simulink model "testmodel4_smith"  (R2018b)
settings: Solver=VariableStepAuto  StartTime=0.0  StopTime=100  RelTol=1e-6
libraries: simulink x5
settings Model: Creator=Khor Jia Wei  LastModifiedBy=Khor Jia Wei
settings SolverCC: ZeroCrossAlgorithm=Adaptive

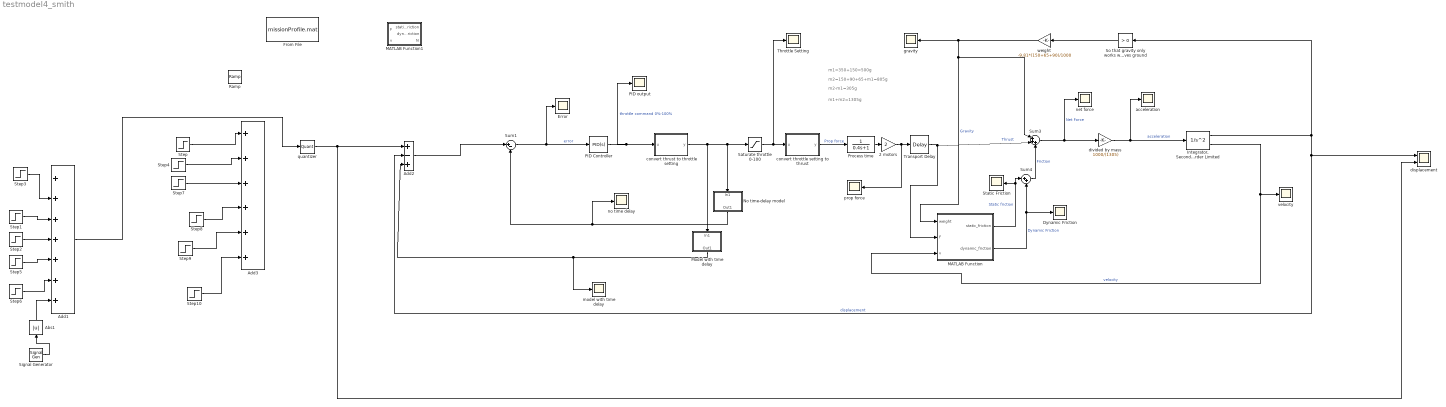
== system testmodel4_smith ==
  note: m1+m2=1305g
  note: m2-m1=305g
  note: m2=150+90+65+m1=805g
  note: m1=350+150=500g
  2 motors : Gain  Gain=2
  Abs1 : Abs
  Add1 : Sum  Inputs=+++++++
  Add2 : Sum  Inputs=+-+
  Add3 : Sum  Inputs=++++++
  Dynamic Friction : Scope
  Error : Scope
  From File : FromFile  FileName=missionProfile.mat  SampleTime=0
  "Integrator, Second-Order Limited" : SecondOrderIntegrator  ICX=0  LimitX=on  LowerLimitX=0  ReinitDXDTwhenXreachesSaturation=on
  MATLAB Function : MATLAB Function  TreatAsAtomicUnit=on
  MATLAB Function1 : MATLAB Function  TreatAsAtomicUnit=on
  Model with time delay : Subsystem
  No time-delay model : Subsystem
  PID Controller : simulink/Continuous/PID Controller  Controller=PID  Form=Parallel  TimeDomain=Continuous-time  SampleTime=-1  IntegratorMethod=Forward Euler  FilterMethod=Forward Euler  ControllerParametersSource=internal  P=20  I=6  D=10  UseFilter=on  N=100  TunerSelectOption=Transfer Function Based (PID Tuner App)  InitialConditionSource=internal  InitialConditionForIntegrator=0  InitialConditionForFilter=0  DifferentiatorICPrevScaledInput=0  ExternalReset=none  TrackingMode=off  Kt=1  LimitOutput=off  UpperSaturationLimit=inf  LowerSaturationLimit=-inf  LinearizeAsGain=on  AntiWindupMode=none  Kb=1  POutMin=[]  POutMax=[]  IOutMin=[]  IOutMax=[]  DOutMin=[]  DOutMax=[]  NOutMin=[]  NOutMax=[]  SumOutMin=[]  SumOutMax=[]  SaturationOutMin=[]  SaturationOutMax=[]  PParamMin=[]  PParamMax=[]  IParamMin=[]  IParamMax=[]  DParamMin=[]  DParamMax=[]  NParamMin=[]  NParamMax=[]  KbParamMin=[]  KbParamMax=[]  KtParamMin=[]  KtParamMax=[]  KbOutMin=[]  KbOutMax=[]  KtOutMin=[]  KtOutMax=[]  IntegratorOutMin=[]  IntegratorOutMax=[]  FilterOutMin=[]  FilterOutMax=[]  SumI1OutMin=[]  SumI1OutMax=[]  SumI2OutMin=[]  SumI2OutMax=[]  SumI3OutMin=[]  SumI3OutMax=[]  SumI4OutMin=[]  SumI4OutMax=[]  SumDOutMin=[]  SumDOutMax=[]  DifferentiatorOutMin=[]  DifferentiatorOutMax=[]  FilterDiffOutCoefMin=[]  FilterDiffOutCoefMax=[]  ReciprocalOutMin=[]  ReciprocalOutMax=[]  SumDenOutMin=[]  SumDenOutMax=[]  SumNumOutMin=[]  SumNumOutMax=[]  DivideOutMin=[]  DivideOutMax=[]  IntegratorContinuousStateAttributes=''  IntegratorStateMustResolveToSignalObject=off  IntegratorRTWStateStorageClass=Auto  FilterContinuousStateAttributes=''  FilterStateMustResolveToSignalObject=off  FilterRTWStateStorageClass=Auto  ParallelPVariant=InternalParameters  IdealPVariant=Disabled  IVariant=InternalParameters  DVariant=InternalParameters  IntegratorVariant=Continuous  SatVariant=Disabled  AWVariant=Passthrough  PCopyVariant=Disabled  TRVariant=Disabled  FdbkBlocksVariant=Forward  IdealPFdbkVariant=Disabled  SatFdbkVariant=Disabled  DerivativeFilterVariant=ContFilter  NVariant=InternalParameters  NCopyVariant=Disabled  FilterICVariant=InternalICsFilter  IntegratorICVariant=InternalICs  ExternalResetVariant=Disabled  TRSumVariant=Passthrough  SumFdbkVariant=Disabled  SumVariant=Sum_PID
  PID output : Scope
  "Process time  " : TransferFcn  Denominator=[0.4 1]
  Ramp : simulink/Sources/Ramp  slope=1  start=0  InitialOutput=0
  Saturate throttle 0-100 : Saturate  UpperLimit=100  LowerLimit=0
  Signal Generator : SignalGenerator  Amplitude=2  Frequency=0.2  Units=rad/sec
  So that gravity only works when the duocopter leaves ground : simulink/Logic and Bit Operations/Compare To Zero  relop=>  OutDataTypeStr=boolean
  Static Friction : Scope
  Step : Step  Time=0.5  After=0.5  SampleTime=0
  Step1 : Step  Time=7  After=0.3  SampleTime=0
  Step10 : Step  Time=32  After=2  SampleTime=0
  Step2 : Step  Time=9  After=0.2  SampleTime=0
  Step3 : Step  Time=5  After=-0.2  SampleTime=0
  Step4 : Step  After=0.5  SampleTime=0
  Step5 : Step  Time=15  After=-0.5  SampleTime=0
  Step6 : Step  Time=25  After=1.4  SampleTime=0
  Step7 : Step  Time=20  SampleTime=0
  Step8 : Step  Time=25  After=-0.5  SampleTime=0
  Step9 : Step  Time=27  After=-1  SampleTime=0
  Sum1 : Sum  Inputs=|+-
  Sum3 : Sum  Inputs=|+++
  Sum4 : Sum  Inputs=|++
  Throttle Setting : Scope
  Transport Delay : TransportDelay  DelayTime=0.6
  acceleration : Scope
  convert throttle setting to thrust : MATLAB Function  TreatAsAtomicUnit=on
  convert thrust to throttle setting : MATLAB Function  TreatAsAtomicUnit=on
  displacement : Scope  NumInputPorts=2
  divided by mass : Gain  Gain=1000/(1305)
  gravity : Scope
  model with time delay : Scope
  net force : Scope
  no time delay : Scope
  prop force : Scope
  quantizer : Quantizer
  velocity : Scope
  weight : Gain  Gain=-9.81*(150+65+90)/1000
  wires:
  So that gravity only works when the duocopter leaves ground/1 -> weight/1
  weight/1 -> MATLAB Function/1(weight), Sum3/1, gravity/1  "Gravity"
  Step5/1 -> Add1/5
  Sum1/1 -> PID Controller/1, Error/1  "error"
  quantizer/1 -> displacement/2, Add2/1
  Step2/1 -> Add1/4
  Step1/1 -> Add1/3
  divided by mass/1 -> "Integrator, Second-Order Limited"/1, acceleration/1  "acceleration"
  "Integrator, Second-Order Limited"/1 -> displacement/1, Add2/2, So that gravity only works when the duocopter leaves ground/1  "displacement"
  "Integrator, Second-Order Limited"/2 -> MATLAB Function/3(v), velocity/1  "velocity"
  PID Controller/1 -> PID output/1, convert thrust to throttle setting/1(u)  "throttle command 0%-100%"
  Sum3/1 -> divided by mass/1, net force/1  "Net Force"
  MATLAB Function/1(static_friction) -> Static Friction/1, Sum4/1  "Static friction"
  MATLAB Function/2(dynamic_friction) -> Dynamic Friction/1, Sum4/2  "Dynamic Friction"
  2 motors/1 -> prop force/1, Transport Delay/1
  Signal Generator/1 -> Abs1/1
  Add2/1 -> Sum1/1
  Model with time delay/1(Out1) -> model with time delay/1, Add2/3
  No time-delay model/1(Out1) -> no time delay/1, Sum1/2
  convert thrust to throttle setting/1(y) -> Saturate throttle 0-100/1, No time-delay model/1(In1), Model with time delay/1(In1)
  Saturate throttle 0-100/1 -> convert throttle setting to thrust/1(u), Throttle Setting/1
  Step6/1 -> Add1/6
  Sum4/1 -> Sum3/3  "Friction"
  Transport Delay/1 -> Sum3/2, MATLAB Function/2(F)  "Thrust"
  Abs1/1 -> Add1/7
  Step/1 -> Add3/1
  Step4/1 -> Add3/2
  Step7/1 -> Add3/3
  Step3/1 -> Add1/2
  Step8/1 -> Add3/4
  Step9/1 -> Add3/5
  Step10/1 -> Add3/6
  Add1/1 -> quantizer/1
  convert throttle setting to thrust/1(y) -> "Process time  "/1  "Prop force"
  "Process time  "/1 -> 2 motors/1

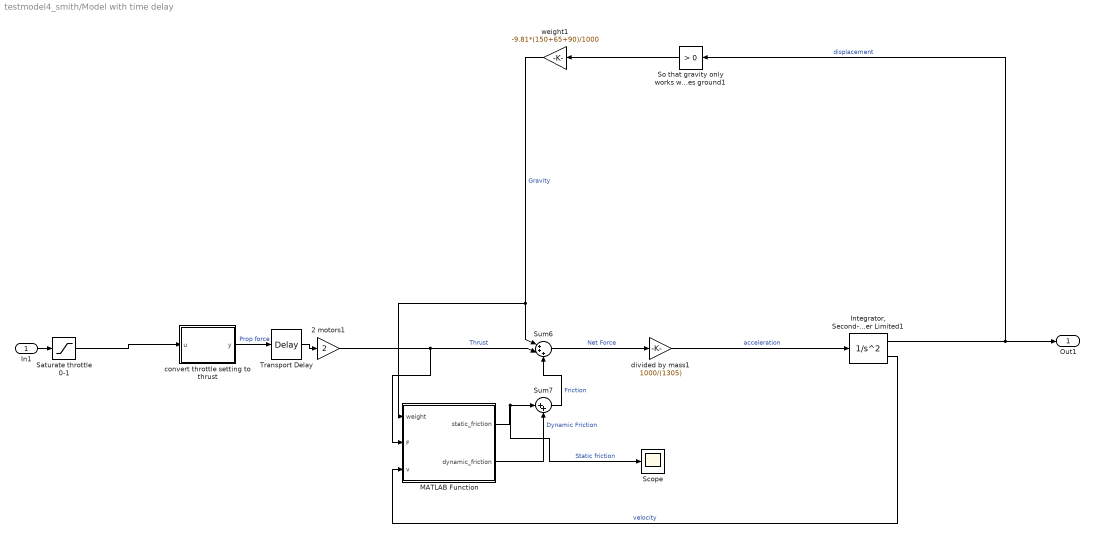
== system testmodel4_smith/Model with time delay ==
  In1 : Inport
  2 motors1 : Gain  Gain=2
  "Integrator, Second-Order Limited1" : SecondOrderIntegrator  ICX=0  LimitX=on  LowerLimitX=0  ReinitDXDTwhenXreachesSaturation=on
  MATLAB Function : MATLAB Function  TreatAsAtomicUnit=on
  Saturate throttle 0-1 : Saturate  UpperLimit=100  LowerLimit=0
  Scope : Scope
  So that gravity only works when the duocopter leaves ground1 : simulink/Logic and Bit Operations/Compare To Zero  relop=>  OutDataTypeStr=boolean
  Sum6 : Sum  Inputs=|+++
  Sum7 : Sum  Inputs=|++
  Transport Delay : TransportDelay  DelayTime=0.8
  convert throttle setting to thrust : MATLAB Function  TreatAsAtomicUnit=on
  divided by mass1 : Gain  Gain=1000/(1305)
  weight1 : Gain  Gain=-9.81*(150+65+90)/1000
  Out1 : Outport
  wires:
  "Integrator, Second-Order Limited1"/2 -> MATLAB Function/3(v)  "velocity"
  divided by mass1/1 -> "Integrator, Second-Order Limited1"/1  "acceleration"
  Transport Delay/1 -> 2 motors1/1
  Saturate throttle 0-1/1 -> convert throttle setting to thrust/1(u)
  So that gravity only works when the duocopter leaves ground1/1 -> weight1/1
  2 motors1/1 -> MATLAB Function/2(F), Sum6/2  "Thrust"
  MATLAB Function/1(static_friction) -> Scope/1, Sum7/1  "Static friction"
  Sum6/1 -> divided by mass1/1  "Net Force"
  "Integrator, Second-Order Limited1"/1 -> Out1/1, So that gravity only works when the duocopter leaves ground1/1  "displacement"
  MATLAB Function/2(dynamic_friction) -> Sum7/2  "Dynamic Friction"
  In1/1 -> Saturate throttle 0-1/1
  convert throttle setting to thrust/1(y) -> Transport Delay/1  "Prop force"
  Sum7/1 -> Sum6/3  "Friction"
  weight1/1 -> MATLAB Function/1(weight), Sum6/1  "Gravity"

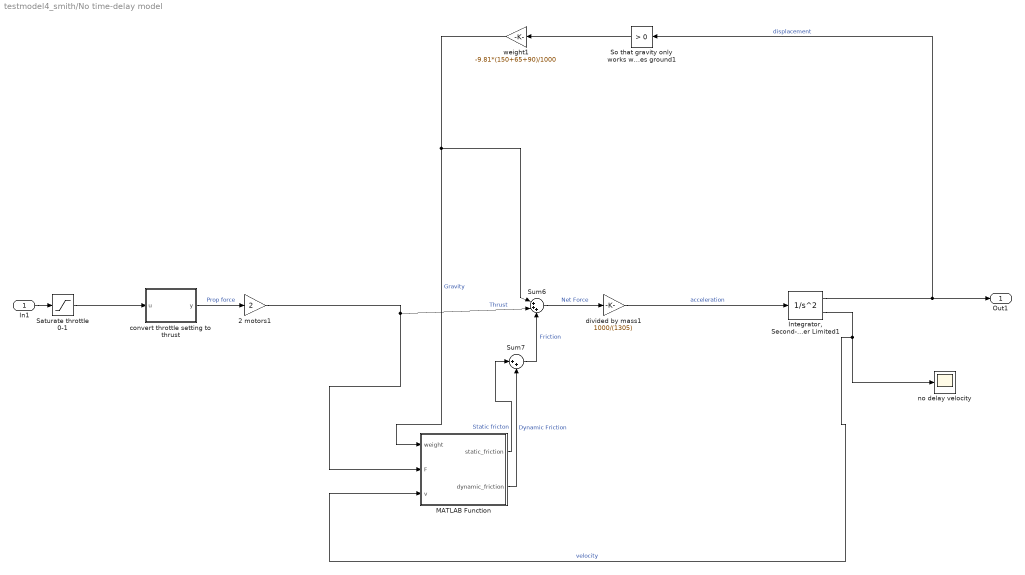
== system testmodel4_smith/No time-delay model ==
  In1 : Inport
  2 motors1 : Gain  Gain=2
  "Integrator, Second-Order Limited1" : SecondOrderIntegrator  ICX=0  LimitX=on  LowerLimitX=0  ReinitDXDTwhenXreachesSaturation=on
  MATLAB Function : MATLAB Function  TreatAsAtomicUnit=on
  Saturate throttle 0-1 : Saturate  UpperLimit=100  LowerLimit=0
  So that gravity only works when the duocopter leaves ground1 : simulink/Logic and Bit Operations/Compare To Zero  relop=>  OutDataTypeStr=boolean
  Sum6 : Sum  Inputs=|+++
  Sum7 : Sum  Inputs=|++
  convert throttle setting to thrust : MATLAB Function  TreatAsAtomicUnit=on
  divided by mass1 : Gain  Gain=1000/(1305)
  no delay velocity : Scope
  weight1 : Gain  Gain=-9.81*(150+65+90)/1000
  Out1 : Outport
  wires:
  divided by mass1/1 -> "Integrator, Second-Order Limited1"/1  "acceleration"
  2 motors1/1 -> MATLAB Function/2(F), Sum6/2  "Thrust"
  weight1/1 -> MATLAB Function/1(weight), Sum6/1  "Gravity"
  So that gravity only works when the duocopter leaves ground1/1 -> weight1/1
  "Integrator, Second-Order Limited1"/1 -> Out1/1, So that gravity only works when the duocopter leaves ground1/1  "displacement"
  "Integrator, Second-Order Limited1"/2 -> MATLAB Function/3(v), no delay velocity/1  "velocity"
  Saturate throttle 0-1/1 -> convert throttle setting to thrust/1(u)
  In1/1 -> Saturate throttle 0-1/1
  Sum6/1 -> divided by mass1/1  "Net Force"
  convert throttle setting to thrust/1(y) -> 2 motors1/1  "Prop force"
  MATLAB Function/2(dynamic_friction) -> Sum7/2  "Dynamic Friction"
  MATLAB Function/1(static_friction) -> Sum7/1  "Static fricton"
  Sum7/1 -> Sum6/3  "Friction"

== matlab function testmodel4_smith/No time-delay model/MATLAB Function ==
  data: weight input; F input; static_friction output; dynamic_friction output; v input
function [static_friction,dynamic_friction]=stickslip(weight,F,v)

%F=T-mg
%v=velocity
weight=double(weight);
%% mass inputs
m_carriage=350/1000; %in kg, given by errikos
m_motorprop=45/1000; %in kg, per motor prop
m_cw=150/1000; %estimated, errikos said 100 to 200g
m_arm=65/1000; 
m_wires=m_cw+150/1000; 
m1=m_carriage+m_cw;
m2=m_arm+2*m_motorprop+m_wires+m_carriage;

%% moment arm lengths

x1=11.5/1000; %in mm, from thrust to edge of arm
x2=10.59/1000; %from cg of arm to edge of arm
h=210.4/1000; %height of carriage
x3=35.8/1000; %thickness of carriage

%% Estimated Tension Force 
tension=m1*(9.81-(F+(m1-m2)*9.81)/(m1+m2));

%% Moment balance to obtain N, and friction
mu_dyn=0.17; %mu_dyn is between 0.11 to 0.17
N2=(F*(x1+x3)-(m2-m1-150/1000)*9.81*(x3+x2)-(m1+150/1000)*9.81*(x3/2)+tension*(x3/2))/h; %Normal contact force on carraige 2
f2=2*mu_dyn*N2; %friction of cart 2
N1=(m_cw*9.81*x3+m_carriage*9.81*(x3/2)-tension*(x3/2))/h; %N of cart 1
f1=2*mu_dyn*N1; %friction of cart 1
max_static_friction=0.130*9.81; 

if abs(v)<1e-5 %we are stuck
    if abs(F+weight)>max_static_friction %we are unstuck
        dynamic_friction=-1*sign(v)*(f1+f2); %dynamic friction
        static_friction=0;
    else
        static_friction=-1*(F+weight); %static friction
        dynamic_friction=0;
    end
else %we are unstuck
    dynamic_friction=-1*sign(v)*(f1+f2);
    static_friction=0;
end

== matlab function testmodel4_smith/MATLAB Function ==
  data: weight input; F input; static_friction output; dynamic_friction output; v input
function [static_friction,dynamic_friction]=stickslip(weight,F,v)

%F=T-mg
%v=velocity
weight=double(weight);
%% mass inputs
m_carriage=350/1000; %in kg, given by errikos
m_motorprop=45/1000; %in kg, per motor prop
m_cw=150/1000; %estimated, errikos said 100 to 200g
m_arm=65/1000; 
m_wires=m_cw+150/1000; 
m1=m_carriage+m_cw;
m2=m_arm+2*m_motorprop+m_wires+m_carriage;

%% moment arm lengths

x1=11.5/1000; %in mm, from thrust to edge of arm
x2=10.59/1000; %from cg of arm to edge of arm
h=210.4/1000; %height of carriage
x3=35.8/1000; %thickness of carriage

%% Estimated Tension Force 
tension=m1*(9.81-(F+(m1-m2)*9.81)/(m1+m2));

%% Moment balance to obtain N, and friction
mu_dyn=0.17; %mu_dyn is between 0.11 to 0.17
N2=(F*(x1+x3)-(m2-m1-150/1000)*9.81*(x3+x2)-(m1+150/1000)*9.81*(x3/2)+tension*(x3/2))/h; %Normal contact force on carraige 2
f2=2*mu_dyn*N2; %friction of cart 2
N1=(m_cw*9.81*(x3)+m_carriage*9.81*(x3/2)-tension*(x3/2))/h; %N of cart 1
f1=2*mu_dyn*N1; %friction of cart 1
max_static_friction=0.130*9.81; 

if abs(v)<1e-5 %we are stuck
    if abs(F+weight)>max_static_friction %we are unstuck
        dynamic_friction=-1*sign(v)*(f1+f2); %dynamic friction
        static_friction=0;
    else
        static_friction=-1*(F+weight); %static friction
        dynamic_friction=0;
    end
else %we are unstuck
    dynamic_friction=-1*sign(v)*(f1+f2);
    static_friction=0;
end

== matlab function testmodel4_smith/convert throttle setting to thrust ==
  data: u input; y output
function y = throttle2thrust(u)
breakpoints1=[0,0.0663455814708608,0.720926457059366,1.46901888630337,2.12359976189187,2.14485238772267,2.45089019968613,2.77150124079070,3.22236051734401,3.63536987932247,3.71329617403539,4.37956599383083,4.38346230856648,5.04371055104320,5.64586828291574,5.86406190811191,5.88410009818094,6.00432923859516,7.26673521294442,7.82780453487743,7.94256871436372,7.96807186536068,8.50363803629673,8.65382325883435,8.80967584826018,10.0253260457817,10.0720818226094,10.0933344484402,10.8201742518534,11.4747551274419,12.3163591103414,12.9709399859299,14.3736132907624,15.0281941663509,15.8631187525608,16.5243790248390,17.2724714540830,17.9270523296715,17.9604493131199,18.7219005357432,18.7619769158813,19.4232371881595,20.8259104929920,21.5856918664429,21.5895881811786,22.1818280209968,22.2285837978245,22.2498364236553,22.2636506304453,22.9766762270685,23.7403539152551,24.3793495319010,24.3949347908436,25.0940449776966,25.1274419611450,25.1486945869758,25.8032754625643,25.8287786135613,26.4299243156324,26.7638941501163,28.0263001244656,28.6808810000541,29.5224849829536,30.1770658585421,30.8103941082998,30.8316467341306,30.8650437175790,31.5797391633746,32.2343200389631,32.2677170224115,33.0759240218626,34.4785973266951,35.9280264083554,36.6293630607716,37.2839439363601,38.0320363656042,38.6866172411927,39.4814654472644,40.1828020996807,41.5854754045132,42.3548204595880,42.3803236105849,42.9146753457592,43.2686833703122,44.4843335678337,45.9337626494940,46.5883435250825,48.0377726067427,48.8326208128145,49.4872016884030,50.1885383408193,50.2041235997618,50.2703609502678,50.2820498944748,50.3154468779232,50.5158287786135,51.6847231993073,53.0406407273120,53.8354889333838,55.8927431138048,55.9139957396356,55.9394988906326,56.5005682125656,56.8559121164565,58.1370204015368,60.2877861356133,60.9423670112019,61.6748741815033,61.6904594404459,61.7060446993884,63.7689662466977,63.8412251745224,64.0750040586612,65.2438984793549,66.0387466854267,66.7400833378429,68.1427566426754,68.7973375182639,69.5921857243357,69.6389415011634,70.2935223767519,71.0416148059960,71.6728177931706,71.6961956815845,71.7174483074152,72.4209102224146,72.4655407366593,73.1923805400725,75.2496347204935,75.9743492613236,75.9977271497375,76.0094160939444,76.0189797755683,77.4939120082255,78.1484928838140,79.5628551328535,79.5979219654743,80.3226365063044,80.3927701715460,80.4395259483738,81.6551761458953,81.7019319227230,81.7231845485538,81.7299853888197,83.1513610043833,84.6007900860436,86.0034633908761,86.7181588366717,86.7515558201201,86.7728084459509,86.7983115969478,87.0788462579143,87.3126251420531,87.3406786081497,87.6866713566751,89.5569024297851,90.3049948590291,90.6322852968234,91.0530872882731,91.8011797175171,92.4713458520482,93.2506087991774,93.9519454515937,95.3546187564262,96.1182964446128,96.7572920612587,97.0845824990529,97.5053844905027,98.2534769197467,98.9080577953352,99.9032879020973,99.9579375113765,100.263975323339];
breakpoints2=[0,0.0164109572459205,0.234387537524814,0.440340894785261,0.434997240110396,0.513532770937965,0.452809422359948,0.524567070851000,0.537639940323439,0.626181329588921,0.548995206507528,0.590408530237738,0.673086742846075,0.703961192078633,0.724445201665616,0.814842026582094,0.658158437722640,0.743147993027647,0.829091772381737,0.912363724398392,0.832208904275407,0.959625381300537,0.981669306242101,0.903457633273616,1.00854950854597,1.04061143659516,0.987174889846509,1.12708148497026,1.15460940299230,1.14422786943785,1.09271206967510,1.26428791519391,1.38530388139737,1.42624518229796,1.51085304798334,1.54710083886118,1.51441548443325,1.64824434706822,1.68658294886249,1.78124197453154,1.66505565431518,1.80475405510095,1.82327872464048,1.93767746513823,1.93834542197259,2.01144661792475,1.94992334043479,2.10059820937305,1.87154973853677,2.09028333656127,2.17762240352491,2.05056217014477,2.21324676802401,2.23911684224360,2.10622523967462,2.32211698498567,2.36292307523010,2.27713312835907,2.36599047180969,2.36405657773689,2.35871292306202,2.39611850578608,2.49453081271486,2.40502459691085,2.75155250612941,2.51786477146177,2.66737259547212,2.62233322035539,2.74003612066043,2.73363391344045,2.85389158959957,2.75147154166465,2.86814133539921,2.75147154166465,3.03599888787343,3.08500465428751,3.05873168546941,3.24433462450975,3.19321366145354,3.26446239045175,3.55552964130238,3.35619512903694,3.59411499194167,3.60289385319323,3.52563351268580,3.66915517116157,3.77976882293129,3.80862455817557,3.74450070207717,3.83213663874497,4.04908901854451,4.12508766280927,3.92217722001646,3.79036707136977,3.99412571331733,4.12924383866750,4.07847911925627,4.13245003147242,4.09940843339950,4.29329403718588,4.28547286988903,4.10573175809809,4.37986124291870,4.38146433932115,4.41780119111025,4.44229294170338,4.57989204958117,4.56421732920156,4.40016713068319,4.64935956035442,4.80594483522094,4.65969062605916,4.80254432770058,4.75177960828935,4.67857153924369,4.83460625574976,4.91253455309155,4.85954331089914,5.03766513339466,4.92366716699752,5.12583543552994,5.12761665375490,5.24205992470827,5.20509964654045,5.32330776510566,5.35427667288045,5.41949354925324,5.45625141625914,5.43309557933472,5.58316321478720,5.46204037549024,5.45834434767345,5.66530166429706,5.66447582675640,5.67534125792863,5.67569750157362,5.72165293177746,5.92471180942235,5.74758746913281,5.88196257202343,5.95570500653658,5.91046206362271,6.09279403828631,6.00807282235026,5.95677373747155,6.06008439451896,6.03514733936958,6.28731694807395,6.34507931051178,6.43478793747771,6.10292269282912,6.30143946400039,6.45106179489662,6.35968529995642,6.40296890282283,6.44749935844671,6.49737346874546,6.49113920495811,6.45106179489662,6.44838996755918,6.44126509465936,6.35220418341160,6.45907727690892,6.46709275892121,6.45373362223406,6.44571814022176,6.44838996755918,6.38604732968576,6.38028805742507,6.44037448554689,6.35541037621653,6.44644682040469,6.40831255749770];

if u<=breakpoints1(153)
    y=2.8E-06*u^3-0.00048*u^2+0.09*u+0.2;
else
    y=breakpoints2(153);
end

== matlab function testmodel4_smith/No time-delay model/convert throttle setting to thrust ==
  data: u input; y output
function y = throttle2thrust(u)
breakpoints1=[0,0.0663455814708608,0.720926457059366,1.46901888630337,2.12359976189187,2.14485238772267,2.45089019968613,2.77150124079070,3.22236051734401,3.63536987932247,3.71329617403539,4.37956599383083,4.38346230856648,5.04371055104320,5.64586828291574,5.86406190811191,5.88410009818094,6.00432923859516,7.26673521294442,7.82780453487743,7.94256871436372,7.96807186536068,8.50363803629673,8.65382325883435,8.80967584826018,10.0253260457817,10.0720818226094,10.0933344484402,10.8201742518534,11.4747551274419,12.3163591103414,12.9709399859299,14.3736132907624,15.0281941663509,15.8631187525608,16.5243790248390,17.2724714540830,17.9270523296715,17.9604493131199,18.7219005357432,18.7619769158813,19.4232371881595,20.8259104929920,21.5856918664429,21.5895881811786,22.1818280209968,22.2285837978245,22.2498364236553,22.2636506304453,22.9766762270685,23.7403539152551,24.3793495319010,24.3949347908436,25.0940449776966,25.1274419611450,25.1486945869758,25.8032754625643,25.8287786135613,26.4299243156324,26.7638941501163,28.0263001244656,28.6808810000541,29.5224849829536,30.1770658585421,30.8103941082998,30.8316467341306,30.8650437175790,31.5797391633746,32.2343200389631,32.2677170224115,33.0759240218626,34.4785973266951,35.9280264083554,36.6293630607716,37.2839439363601,38.0320363656042,38.6866172411927,39.4814654472644,40.1828020996807,41.5854754045132,42.3548204595880,42.3803236105849,42.9146753457592,43.2686833703122,44.4843335678337,45.9337626494940,46.5883435250825,48.0377726067427,48.8326208128145,49.4872016884030,50.1885383408193,50.2041235997618,50.2703609502678,50.2820498944748,50.3154468779232,50.5158287786135,51.6847231993073,53.0406407273120,53.8354889333838,55.8927431138048,55.9139957396356,55.9394988906326,56.5005682125656,56.8559121164565,58.1370204015368,60.2877861356133,60.9423670112019,61.6748741815033,61.6904594404459,61.7060446993884,63.7689662466977,63.8412251745224,64.0750040586612,65.2438984793549,66.0387466854267,66.7400833378429,68.1427566426754,68.7973375182639,69.5921857243357,69.6389415011634,70.2935223767519,71.0416148059960,71.6728177931706,71.6961956815845,71.7174483074152,72.4209102224146,72.4655407366593,73.1923805400725,75.2496347204935,75.9743492613236,75.9977271497375,76.0094160939444,76.0189797755683,77.4939120082255,78.1484928838140,79.5628551328535,79.5979219654743,80.3226365063044,80.3927701715460,80.4395259483738,81.6551761458953,81.7019319227230,81.7231845485538,81.7299853888197,83.1513610043833,84.6007900860436,86.0034633908761,86.7181588366717,86.7515558201201,86.7728084459509,86.7983115969478,87.0788462579143,87.3126251420531,87.3406786081497,87.6866713566751,89.5569024297851,90.3049948590291,90.6322852968234,91.0530872882731,91.8011797175171,92.4713458520482,93.2506087991774,93.9519454515937,95.3546187564262,96.1182964446128,96.7572920612587,97.0845824990529,97.5053844905027,98.2534769197467,98.9080577953352,99.9032879020973,99.9579375113765,100.263975323339];
breakpoints2=[0,0.0164109572459205,0.234387537524814,0.440340894785261,0.434997240110396,0.513532770937965,0.452809422359948,0.524567070851000,0.537639940323439,0.626181329588921,0.548995206507528,0.590408530237738,0.673086742846075,0.703961192078633,0.724445201665616,0.814842026582094,0.658158437722640,0.743147993027647,0.829091772381737,0.912363724398392,0.832208904275407,0.959625381300537,0.981669306242101,0.903457633273616,1.00854950854597,1.04061143659516,0.987174889846509,1.12708148497026,1.15460940299230,1.14422786943785,1.09271206967510,1.26428791519391,1.38530388139737,1.42624518229796,1.51085304798334,1.54710083886118,1.51441548443325,1.64824434706822,1.68658294886249,1.78124197453154,1.66505565431518,1.80475405510095,1.82327872464048,1.93767746513823,1.93834542197259,2.01144661792475,1.94992334043479,2.10059820937305,1.87154973853677,2.09028333656127,2.17762240352491,2.05056217014477,2.21324676802401,2.23911684224360,2.10622523967462,2.32211698498567,2.36292307523010,2.27713312835907,2.36599047180969,2.36405657773689,2.35871292306202,2.39611850578608,2.49453081271486,2.40502459691085,2.75155250612941,2.51786477146177,2.66737259547212,2.62233322035539,2.74003612066043,2.73363391344045,2.85389158959957,2.75147154166465,2.86814133539921,2.75147154166465,3.03599888787343,3.08500465428751,3.05873168546941,3.24433462450975,3.19321366145354,3.26446239045175,3.55552964130238,3.35619512903694,3.59411499194167,3.60289385319323,3.52563351268580,3.66915517116157,3.77976882293129,3.80862455817557,3.74450070207717,3.83213663874497,4.04908901854451,4.12508766280927,3.92217722001646,3.79036707136977,3.99412571331733,4.12924383866750,4.07847911925627,4.13245003147242,4.09940843339950,4.29329403718588,4.28547286988903,4.10573175809809,4.37986124291870,4.38146433932115,4.41780119111025,4.44229294170338,4.57989204958117,4.56421732920156,4.40016713068319,4.64935956035442,4.80594483522094,4.65969062605916,4.80254432770058,4.75177960828935,4.67857153924369,4.83460625574976,4.91253455309155,4.85954331089914,5.03766513339466,4.92366716699752,5.12583543552994,5.12761665375490,5.24205992470827,5.20509964654045,5.32330776510566,5.35427667288045,5.41949354925324,5.45625141625914,5.43309557933472,5.58316321478720,5.46204037549024,5.45834434767345,5.66530166429706,5.66447582675640,5.67534125792863,5.67569750157362,5.72165293177746,5.92471180942235,5.74758746913281,5.88196257202343,5.95570500653658,5.91046206362271,6.09279403828631,6.00807282235026,5.95677373747155,6.06008439451896,6.03514733936958,6.28731694807395,6.34507931051178,6.43478793747771,6.10292269282912,6.30143946400039,6.45106179489662,6.35968529995642,6.40296890282283,6.44749935844671,6.49737346874546,6.49113920495811,6.45106179489662,6.44838996755918,6.44126509465936,6.35220418341160,6.45907727690892,6.46709275892121,6.45373362223406,6.44571814022176,6.44838996755918,6.38604732968576,6.38028805742507,6.44037448554689,6.35541037621653,6.44644682040469,6.40831255749770];

if u<=breakpoints1(153)
    y=2.8E-06*u^3-0.00048*u^2+0.09*u+0.2;
else
    y=breakpoints2(153);
end

== matlab function testmodel4_smith/Model with time delay/convert throttle setting to thrust ==
  data: u input; y output
function y = throttle2thrust(u)
breakpoints1=[0,0.0663455814708608,0.720926457059366,1.46901888630337,2.12359976189187,2.14485238772267,2.45089019968613,2.77150124079070,3.22236051734401,3.63536987932247,3.71329617403539,4.37956599383083,4.38346230856648,5.04371055104320,5.64586828291574,5.86406190811191,5.88410009818094,6.00432923859516,7.26673521294442,7.82780453487743,7.94256871436372,7.96807186536068,8.50363803629673,8.65382325883435,8.80967584826018,10.0253260457817,10.0720818226094,10.0933344484402,10.8201742518534,11.4747551274419,12.3163591103414,12.9709399859299,14.3736132907624,15.0281941663509,15.8631187525608,16.5243790248390,17.2724714540830,17.9270523296715,17.9604493131199,18.7219005357432,18.7619769158813,19.4232371881595,20.8259104929920,21.5856918664429,21.5895881811786,22.1818280209968,22.2285837978245,22.2498364236553,22.2636506304453,22.9766762270685,23.7403539152551,24.3793495319010,24.3949347908436,25.0940449776966,25.1274419611450,25.1486945869758,25.8032754625643,25.8287786135613,26.4299243156324,26.7638941501163,28.0263001244656,28.6808810000541,29.5224849829536,30.1770658585421,30.8103941082998,30.8316467341306,30.8650437175790,31.5797391633746,32.2343200389631,32.2677170224115,33.0759240218626,34.4785973266951,35.9280264083554,36.6293630607716,37.2839439363601,38.0320363656042,38.6866172411927,39.4814654472644,40.1828020996807,41.5854754045132,42.3548204595880,42.3803236105849,42.9146753457592,43.2686833703122,44.4843335678337,45.9337626494940,46.5883435250825,48.0377726067427,48.8326208128145,49.4872016884030,50.1885383408193,50.2041235997618,50.2703609502678,50.2820498944748,50.3154468779232,50.5158287786135,51.6847231993073,53.0406407273120,53.8354889333838,55.8927431138048,55.9139957396356,55.9394988906326,56.5005682125656,56.8559121164565,58.1370204015368,60.2877861356133,60.9423670112019,61.6748741815033,61.6904594404459,61.7060446993884,63.7689662466977,63.8412251745224,64.0750040586612,65.2438984793549,66.0387466854267,66.7400833378429,68.1427566426754,68.7973375182639,69.5921857243357,69.6389415011634,70.2935223767519,71.0416148059960,71.6728177931706,71.6961956815845,71.7174483074152,72.4209102224146,72.4655407366593,73.1923805400725,75.2496347204935,75.9743492613236,75.9977271497375,76.0094160939444,76.0189797755683,77.4939120082255,78.1484928838140,79.5628551328535,79.5979219654743,80.3226365063044,80.3927701715460,80.4395259483738,81.6551761458953,81.7019319227230,81.7231845485538,81.7299853888197,83.1513610043833,84.6007900860436,86.0034633908761,86.7181588366717,86.7515558201201,86.7728084459509,86.7983115969478,87.0788462579143,87.3126251420531,87.3406786081497,87.6866713566751,89.5569024297851,90.3049948590291,90.6322852968234,91.0530872882731,91.8011797175171,92.4713458520482,93.2506087991774,93.9519454515937,95.3546187564262,96.1182964446128,96.7572920612587,97.0845824990529,97.5053844905027,98.2534769197467,98.9080577953352,99.9032879020973,99.9579375113765,100.263975323339];
breakpoints2=[0,0.0164109572459205,0.234387537524814,0.440340894785261,0.434997240110396,0.513532770937965,0.452809422359948,0.524567070851000,0.537639940323439,0.626181329588921,0.548995206507528,0.590408530237738,0.673086742846075,0.703961192078633,0.724445201665616,0.814842026582094,0.658158437722640,0.743147993027647,0.829091772381737,0.912363724398392,0.832208904275407,0.959625381300537,0.981669306242101,0.903457633273616,1.00854950854597,1.04061143659516,0.987174889846509,1.12708148497026,1.15460940299230,1.14422786943785,1.09271206967510,1.26428791519391,1.38530388139737,1.42624518229796,1.51085304798334,1.54710083886118,1.51441548443325,1.64824434706822,1.68658294886249,1.78124197453154,1.66505565431518,1.80475405510095,1.82327872464048,1.93767746513823,1.93834542197259,2.01144661792475,1.94992334043479,2.10059820937305,1.87154973853677,2.09028333656127,2.17762240352491,2.05056217014477,2.21324676802401,2.23911684224360,2.10622523967462,2.32211698498567,2.36292307523010,2.27713312835907,2.36599047180969,2.36405657773689,2.35871292306202,2.39611850578608,2.49453081271486,2.40502459691085,2.75155250612941,2.51786477146177,2.66737259547212,2.62233322035539,2.74003612066043,2.73363391344045,2.85389158959957,2.75147154166465,2.86814133539921,2.75147154166465,3.03599888787343,3.08500465428751,3.05873168546941,3.24433462450975,3.19321366145354,3.26446239045175,3.55552964130238,3.35619512903694,3.59411499194167,3.60289385319323,3.52563351268580,3.66915517116157,3.77976882293129,3.80862455817557,3.74450070207717,3.83213663874497,4.04908901854451,4.12508766280927,3.92217722001646,3.79036707136977,3.99412571331733,4.12924383866750,4.07847911925627,4.13245003147242,4.09940843339950,4.29329403718588,4.28547286988903,4.10573175809809,4.37986124291870,4.38146433932115,4.41780119111025,4.44229294170338,4.57989204958117,4.56421732920156,4.40016713068319,4.64935956035442,4.80594483522094,4.65969062605916,4.80254432770058,4.75177960828935,4.67857153924369,4.83460625574976,4.91253455309155,4.85954331089914,5.03766513339466,4.92366716699752,5.12583543552994,5.12761665375490,5.24205992470827,5.20509964654045,5.32330776510566,5.35427667288045,5.41949354925324,5.45625141625914,5.43309557933472,5.58316321478720,5.46204037549024,5.45834434767345,5.66530166429706,5.66447582675640,5.67534125792863,5.67569750157362,5.72165293177746,5.92471180942235,5.74758746913281,5.88196257202343,5.95570500653658,5.91046206362271,6.09279403828631,6.00807282235026,5.95677373747155,6.06008439451896,6.03514733936958,6.28731694807395,6.34507931051178,6.43478793747771,6.10292269282912,6.30143946400039,6.45106179489662,6.35968529995642,6.40296890282283,6.44749935844671,6.49737346874546,6.49113920495811,6.45106179489662,6.44838996755918,6.44126509465936,6.35220418341160,6.45907727690892,6.46709275892121,6.45373362223406,6.44571814022176,6.44838996755918,6.38604732968576,6.38028805742507,6.44037448554689,6.35541037621653,6.44644682040469,6.40831255749770];

if u<=breakpoints1(153)
    y=2.8E-06*u^3-0.00048*u^2+0.09*u+0.2;
else
    y=breakpoints2(153);
end

== matlab function testmodel4_smith/convert thrust to throttle setting ==
  data: u input; y output
function y = thrust2throttle(u)
breakpoints1=[0,0.0663455814708608,0.720926457059366,1.46901888630337,2.12359976189187,2.14485238772267,2.45089019968613,2.77150124079070,3.22236051734401,3.63536987932247,3.71329617403539,4.37956599383083,4.38346230856648,5.04371055104320,5.64586828291574,5.86406190811191,5.88410009818094,6.00432923859516,7.26673521294442,7.82780453487743,7.94256871436372,7.96807186536068,8.50363803629673,8.65382325883435,8.80967584826018,10.0253260457817,10.0720818226094,10.0933344484402,10.8201742518534,11.4747551274419,12.3163591103414,12.9709399859299,14.3736132907624,15.0281941663509,15.8631187525608,16.5243790248390,17.2724714540830,17.9270523296715,17.9604493131199,18.7219005357432,18.7619769158813,19.4232371881595,20.8259104929920,21.5856918664429,21.5895881811786,22.1818280209968,22.2285837978245,22.2498364236553,22.2636506304453,22.9766762270685,23.7403539152551,24.3793495319010,24.3949347908436,25.0940449776966,25.1274419611450,25.1486945869758,25.8032754625643,25.8287786135613,26.4299243156324,26.7638941501163,28.0263001244656,28.6808810000541,29.5224849829536,30.1770658585421,30.8103941082998,30.8316467341306,30.8650437175790,31.5797391633746,32.2343200389631,32.2677170224115,33.0759240218626,34.4785973266951,35.9280264083554,36.6293630607716,37.2839439363601,38.0320363656042,38.6866172411927,39.4814654472644,40.1828020996807,41.5854754045132,42.3548204595880,42.3803236105849,42.9146753457592,43.2686833703122,44.4843335678337,45.9337626494940,46.5883435250825,48.0377726067427,48.8326208128145,49.4872016884030,50.1885383408193,50.2041235997618,50.2703609502678,50.2820498944748,50.3154468779232,50.5158287786135,51.6847231993073,53.0406407273120,53.8354889333838,55.8927431138048,55.9139957396356,55.9394988906326,56.5005682125656,56.8559121164565,58.1370204015368,60.2877861356133,60.9423670112019,61.6748741815033,61.6904594404459,61.7060446993884,63.7689662466977,63.8412251745224,64.0750040586612,65.2438984793549,66.0387466854267,66.7400833378429,68.1427566426754,68.7973375182639,69.5921857243357,69.6389415011634,70.2935223767519,71.0416148059960,71.6728177931706,71.6961956815845,71.7174483074152,72.4209102224146,72.4655407366593,73.1923805400725,75.2496347204935,75.9743492613236,75.9977271497375,76.0094160939444,76.0189797755683,77.4939120082255,78.1484928838140,79.5628551328535,79.5979219654743,80.3226365063044,80.3927701715460,80.4395259483738,81.6551761458953,81.7019319227230,81.7231845485538,81.7299853888197,83.1513610043833,84.6007900860436,86.0034633908761,86.7181588366717,86.7515558201201,86.7728084459509,86.7983115969478,87.0788462579143,87.3126251420531,87.3406786081497,87.6866713566751,89.5569024297851,90.3049948590291,90.6322852968234,91.0530872882731,91.8011797175171,92.4713458520482,93.2506087991774,93.9519454515937,95.3546187564262,96.1182964446128,96.7572920612587,97.0845824990529,97.5053844905027,98.2534769197467,98.9080577953352,99.9032879020973,99.9579375113765,100.263975323339];
breakpoints2=[0,0.0164109572459205,0.234387537524814,0.440340894785261,0.434997240110396,0.513532770937965,0.452809422359948,0.524567070851000,0.537639940323439,0.626181329588921,0.548995206507528,0.590408530237738,0.673086742846075,0.703961192078633,0.724445201665616,0.814842026582094,0.658158437722640,0.743147993027647,0.829091772381737,0.912363724398392,0.832208904275407,0.959625381300537,0.981669306242101,0.903457633273616,1.00854950854597,1.04061143659516,0.987174889846509,1.12708148497026,1.15460940299230,1.14422786943785,1.09271206967510,1.26428791519391,1.38530388139737,1.42624518229796,1.51085304798334,1.54710083886118,1.51441548443325,1.64824434706822,1.68658294886249,1.78124197453154,1.66505565431518,1.80475405510095,1.82327872464048,1.93767746513823,1.93834542197259,2.01144661792475,1.94992334043479,2.10059820937305,1.87154973853677,2.09028333656127,2.17762240352491,2.05056217014477,2.21324676802401,2.23911684224360,2.10622523967462,2.32211698498567,2.36292307523010,2.27713312835907,2.36599047180969,2.36405657773689,2.35871292306202,2.39611850578608,2.49453081271486,2.40502459691085,2.75155250612941,2.51786477146177,2.66737259547212,2.62233322035539,2.74003612066043,2.73363391344045,2.85389158959957,2.75147154166465,2.86814133539921,2.75147154166465,3.03599888787343,3.08500465428751,3.05873168546941,3.24433462450975,3.19321366145354,3.26446239045175,3.55552964130238,3.35619512903694,3.59411499194167,3.60289385319323,3.52563351268580,3.66915517116157,3.77976882293129,3.80862455817557,3.74450070207717,3.83213663874497,4.04908901854451,4.12508766280927,3.92217722001646,3.79036707136977,3.99412571331733,4.12924383866750,4.07847911925627,4.13245003147242,4.09940843339950,4.29329403718588,4.28547286988903,4.10573175809809,4.37986124291870,4.38146433932115,4.41780119111025,4.44229294170338,4.57989204958117,4.56421732920156,4.40016713068319,4.64935956035442,4.80594483522094,4.65969062605916,4.80254432770058,4.75177960828935,4.67857153924369,4.83460625574976,4.91253455309155,4.85954331089914,5.03766513339466,4.92366716699752,5.12583543552994,5.12761665375490,5.24205992470827,5.20509964654045,5.32330776510566,5.35427667288045,5.41949354925324,5.45625141625914,5.43309557933472,5.58316321478720,5.46204037549024,5.45834434767345,5.66530166429706,5.66447582675640,5.67534125792863,5.67569750157362,5.72165293177746,5.92471180942235,5.74758746913281,5.88196257202343,5.95570500653658,5.91046206362271,6.09279403828631,6.00807282235026,5.95677373747155,6.06008439451896,6.03514733936958,6.28731694807395,6.34507931051178,6.43478793747771,6.10292269282912,6.30143946400039,6.45106179489662,6.35968529995642,6.40296890282283,6.44749935844671,6.49737346874546,6.49113920495811,6.45106179489662,6.44838996755918,6.44126509465936,6.35220418341160,6.45907727690892,6.46709275892121,6.45373362223406,6.44571814022176,6.44838996755918,6.38604732968576,6.38028805742507,6.44037448554689,6.35541037621653,6.44644682040469,6.40831255749770];

if u/2<=0
    y=0;
elseif u/2<=breakpoints2(153)
    y=-0.00056*(u/2)^7+0.024*(u/2)^6-0.36*(u/2)^5+2.5*(u/2)^4-8.7*(u/2)^3+15*(u/2)^2+0.39*(u/2)-0.18;
else
    y=100;
end

== matlab function testmodel4_smith/MATLAB Function1 ==
  data: F input; static_friction output; dynamic_friction output; N output; v input
function [static_friction,dynamic_friction,N]=stickslip(F,v)

%u(1) is the net thrust-mg
%u(2) is the velocity

%input
delta=0.1; %moment arm of T and mg
l=0.2104; %height of cart
m=(150+65+90)/1000;
mu_dyn=0.17; %mu_dyn is between 0.11 to 0.17
max_static_friction=0.130*9.81; 

N=abs((F-m*9.81)*delta/l); %normal contact force, obtained using balance of moment
%N=0.2;
if abs(v)<1e-5 %we are stuck
    if abs(F)>max_static_friction %we are unstuck
        dynamic_friction=-1*sign(v)*(2*N*mu_dyn); %dynamic friction
        static_friction=0;
    else
        static_friction=-1*F; %static friction
        dynamic_friction=0;
    end
else %we are unstuck
    dynamic_friction=-1*sign(v)*(2*N*mu_dyn);
    static_friction=0;
end

== matlab function testmodel4_smith/Model with time delay/MATLAB Function ==
  data: weight input; F input; static_friction output; dynamic_friction output; v input
function [static_friction,dynamic_friction]=stickslip(weight,F,v)

%F=T-mg
%v=velocity
weight=double(weight);
%% mass inputs
m_carriage=350/1000; %in kg, given by errikos
m_motorprop=45/1000; %in kg, per motor prop
m_cw=150/1000; %estimated, errikos said 100 to 200g
m_arm=65/1000; 
m_wires=m_cw+150/1000; 
m1=m_carriage+m_cw;
m2=m_arm+2*m_motorprop+m_wires+m_carriage;

%% moment arm lengths

x1=11.5/1000; %in mm, from thrust to edge of arm
x2=10.59/1000; %from cg of arm to edge of arm
h=210.4/1000; %height of carriage
x3=35.8/1000; %thickness of carriage

%% Estimated Tension Force 
tension=m1*(9.81-(F+(m1-m2)*9.81)/(m1+m2));

%% Moment balance to obtain N, and friction
mu_dyn=0.17; %mu_dyn is between 0.11 to 0.17
N2=(F*(x1+x3)-(m2-m1-150/1000)*9.81*(x3+x2)-(m1+150/1000)*9.81*(x3/2)+tension*(x3/2))/h; %Normal contact force on carraige 2
f2=2*mu_dyn*N2; %friction of cart 2
N1=(m_cw*9.81*x3+m_carriage*9.81*(x3/2)-tension*(x3/2))/h; %N of cart 1
f1=2*mu_dyn*N1; %friction of cart 1
max_static_friction=0.130*9.81; 

if abs(v)<1e-5 %we are stuck
    if abs(F+weight)>max_static_friction %we are unstuck
        dynamic_friction=-1*sign(v)*(f1+f2); %dynamic friction
        static_friction=0;
    else
        static_friction=-1*(F+weight); %static friction
        dynamic_friction=0;
    end
else %we are unstuck
    dynamic_friction=-1*sign(v)*(f1+f2);
    static_friction=0;
end
